simulink model "Aufgabe4_bode"  (R2025b)
settings: Solver=VariableStepAuto  StartTime=0.0  StopTime=10.0  RelTol=1e-3
settings Model: Creator=henri  LastModifiedBy=henri

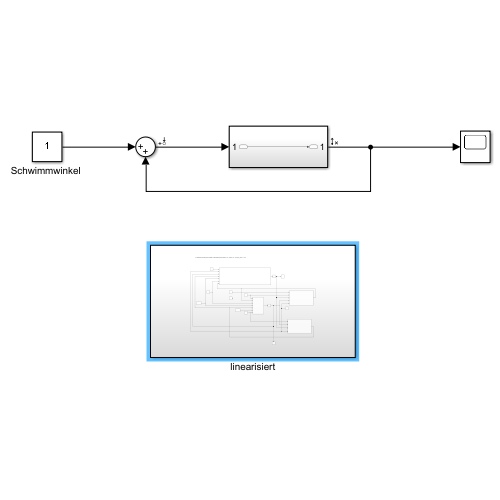
[thumbnail: Simulink's stored preview of the top-level diagram]
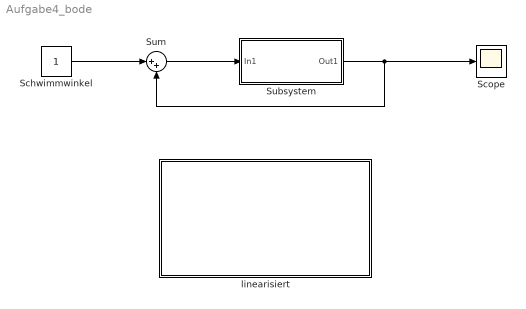
== system Aufgabe4_bode ==
  "Schwimmwinkel " : Constant
  Scope : Scope
  Subsystem : Subsystem
  Sum : Sum  Inputs=|++
  linearisiert : Subsystem
  wires:
  Sum/1 -> Subsystem/1(In1)
  Subsystem/1(Out1) -> Sum/2, Scope/1
  "Schwimmwinkel "/1 -> Sum/1

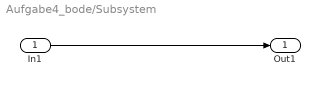
== system Aufgabe4_bode/Subsystem ==
  In1 : Inport
  Out1 : Outport
  wires:
  In1/1 -> Out1/1

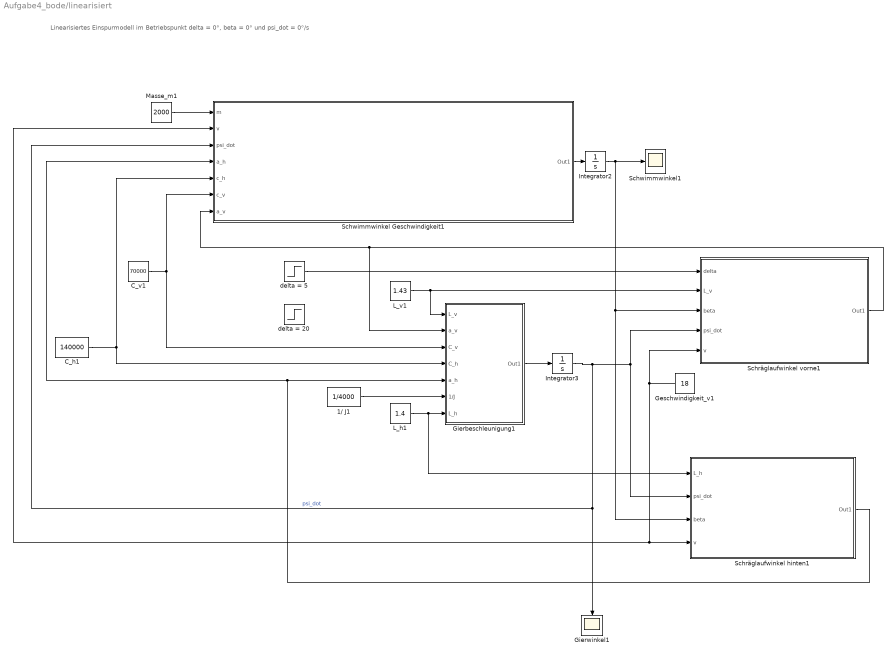
== system Aufgabe4_bode/linearisiert ==
  note: Linearisiertes Einspurmodell im Betriebspunkt delta = 0°, beta = 0° und psi_dot = 0°/s
  1/ J1 : Constant  Value=1/4000
  C_h1 : Constant  Value=140000
  C_v1 : Constant  Value=70000
  Geschwindigkeit_v1 : Constant  Value=18
  Gierbeschleunigung1 : Subsystem
  Gierwinkel1 : Scope
      settings: ActiveDisplayYMinimum=10.3809891207316  ActiveDisplayYMaximum=19.349294137123358  DataLoggingVariableName=ScopeData2
  Integrator2 : Integrator
  Integrator3 : Integrator
  L_h1 : Constant  Value=1.4
  L_v1 : Constant  Value=1.43
  Masse_m1 : Constant  Value=2000
  Schräglaufwinkel hinten1 : Subsystem
  Schräglaufwinkel vorne1 : Subsystem
  Schwimmwinkel Geschwindigkeit1 : Subsystem
  Schwimmwinkel1 : Scope
      settings: ActiveDisplayYMinimum=-2.8333418536826671  ActiveDisplayYMaximum=18.290047988702511  DataLoggingVariableName=ScopeData3
  delta = 20 : Step  After=20  SampleTime=0
  delta = 5 : Step  After=5  SampleTime=0
  wires:
  Integrator3/1 -> Schwimmwinkel Geschwindigkeit1/3(psi_dot), Gierwinkel1/1, Schräglaufwinkel hinten1/2(psi_dot), Schräglaufwinkel vorne1/4(psi_dot)  "psi_dot"
  Schräglaufwinkel hinten1/1(Out1) -> Schwimmwinkel Geschwindigkeit1/4(a_h), Gierbeschleunigung1/5(a_h)
  Integrator2/1 -> Schwimmwinkel1/1, Schräglaufwinkel vorne1/3(beta), Schräglaufwinkel hinten1/3(beta)
  C_v1/1 -> Schwimmwinkel Geschwindigkeit1/6(c_v), Gierbeschleunigung1/3(C_v)
  Geschwindigkeit_v1/1 -> Schwimmwinkel Geschwindigkeit1/2(v), Schräglaufwinkel hinten1/4(v), Schräglaufwinkel vorne1/5(v)
  L_v1/1 -> Gierbeschleunigung1/1(L_v), Schräglaufwinkel vorne1/2(L_v)
  C_h1/1 -> Gierbeschleunigung1/4(C_h), Schwimmwinkel Geschwindigkeit1/5(c_h)
  Schräglaufwinkel vorne1/1(Out1) -> Gierbeschleunigung1/2(a_v), Schwimmwinkel Geschwindigkeit1/7(a_v)
  Gierbeschleunigung1/1(Out1) -> Integrator3/1
  delta = 5/1 -> Schräglaufwinkel vorne1/1(delta)
  Schwimmwinkel Geschwindigkeit1/1(Out1) -> Integrator2/1
  1/ J1/1 -> Gierbeschleunigung1/6(1/J)
  L_h1/1 -> Schräglaufwinkel hinten1/1(L_h), Gierbeschleunigung1/7(L_h)
  Masse_m1/1 -> Schwimmwinkel Geschwindigkeit1/1(m)

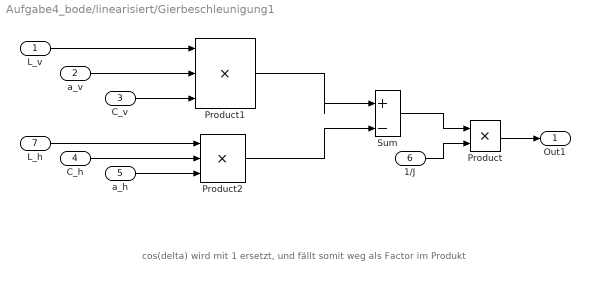
== system Aufgabe4_bode/linearisiert/Gierbeschleunigung1 ==
  note: cos(delta) wird mit 1 ersetzt, und fällt somit weg als Factor im Produkt
  L_v : Inport
  a_v : Inport  Port=2
  C_v : Inport  Port=3
  C_h : Inport  Port=4
  a_h : Inport  Port=5
  1/J : Inport  Port=6
  L_h : Inport  Port=7
  Product : Product
  Product1 : Product  Inputs=3
  Product2 : Product  Inputs=3
  Sum : Sum  Inputs=|+-
  Out1 : Outport
  wires:
  Product1/1 -> Sum/1
  Product2/1 -> Sum/2
  a_v/1 -> Product1/2
  1/J/1 -> Product/2
  Sum/1 -> Product/1
  Product/1 -> Out1/1
  a_h/1 -> Product2/3
  C_h/1 -> Product2/2
  L_h/1 -> Product2/1
  L_v/1 -> Product1/1
  C_v/1 -> Product1/3

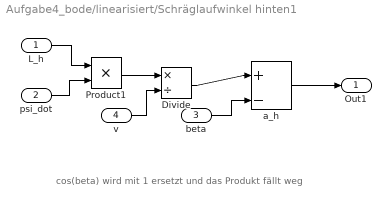
== system Aufgabe4_bode/linearisiert/Schräglaufwinkel hinten1 ==
  note: cos(beta) wird mit 1 ersetzt und das Produkt fällt weg
  L_h : Inport
  psi_dot : Inport  Port=2
  beta : Inport  Port=3
  v : Inport  Port=4
  Divide : Product  Inputs=*/
  Product1 : Product
  a_h : Sum  Inputs=|+-
  Out1 : Outport
  wires:
  L_h/1 -> Product1/1
  psi_dot/1 -> Product1/2
  v/1 -> Divide/2
  Product1/1 -> Divide/1
  Divide/1 -> a_h/1
  a_h/1 -> Out1/1
  beta/1 -> a_h/2

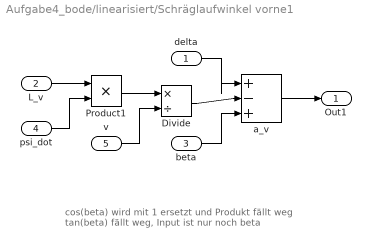
== system Aufgabe4_bode/linearisiert/Schräglaufwinkel vorne1 ==
  note: cos(beta) wird mit 1 ersetzt und Produkt fällt weg
      | tan(beta) fällt weg, Input ist nur noch beta
  delta : Inport
  L_v : Inport  Port=2
  beta : Inport  Port=3
  psi_dot : Inport  Port=4
  v : Inport  Port=5
  Divide : Product  Inputs=*/
  Product1 : Product
  a_v : Sum  Inputs=|+-+
  Out1 : Outport
  wires:
  a_v/1 -> Out1/1
  beta/1 -> a_v/3
  Divide/1 -> a_v/2
  delta/1 -> a_v/1
  v/1 -> Divide/2
  Product1/1 -> Divide/1
  psi_dot/1 -> Product1/2
  L_v/1 -> Product1/1

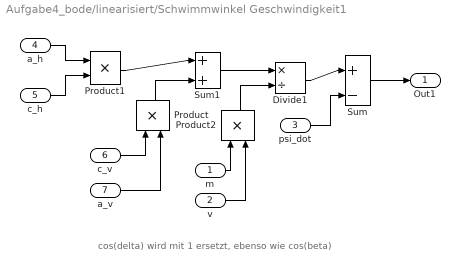
== system Aufgabe4_bode/linearisiert/Schwimmwinkel Geschwindigkeit1 ==
  note: cos(delta) wird mit 1 ersetzt, ebenso wie cos(beta)
  m : Inport
  v : Inport  Port=2
  psi_dot : Inport  Port=3
  a_h : Inport  Port=4
  c_h : Inport  Port=5
  c_v : Inport  Port=6
  a_v : Inport  Port=7
  Divide1 : Product  Inputs=*/
  Product : Product
  Product1 : Product
  Product2 : Product
  Sum : Sum  Inputs=|+-
  Sum1 : Sum  Inputs=|++
  Out1 : Outport
  wires:
  c_v/1 -> Product/1
  v/1 -> Product2/2
  c_h/1 -> Product1/2
  Divide1/1 -> Sum/1
  m/1 -> Product2/1
  a_h/1 -> Product1/1
  Product1/1 -> Sum1/1
  psi_dot/1 -> Sum/2
  Product/1 -> Sum1/2
  Product2/1 -> Divide1/2
  Sum1/1 -> Divide1/1
  Sum/1 -> Out1/1
  a_v/1 -> Product/2
